simulink model "Model_sim"  (R2024b)
settings: Solver=FixedStepAuto  StartTime=0.0  StopTime=10  FixedStep=0.001  RelTol=1e-3
values from neighbouring files (symbols this model uses):
  A = [      0             1            0         0 ... (first row only)    [QuarterCarModel.m]
  A_Nodamp = [      0             1            0         0 ... (first row only)    [QuarterCarModel.m]
  B = [  0     0     0 ... (first row only)    [QuarterCarModel.m]
  C = [1 0 0 0 ... (first row only)    [QuarterCarModel.m]
  D = zeros(4,3)    [QuarterCarModel.m]
undefined symbols (not defined in the file or in its folder): A_sky, B_sky, c_sky, C_sky, D_sky
settings Model: Creator=elija  LastModifiedBy=elija

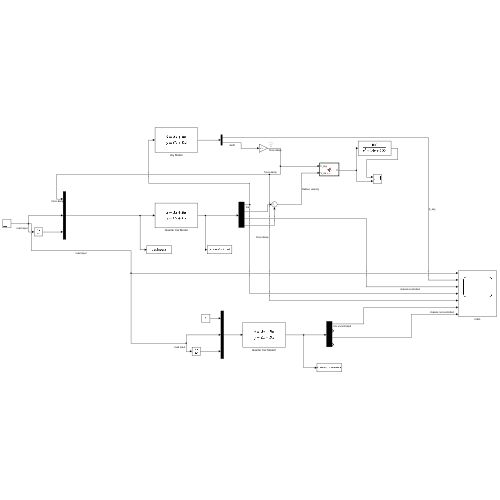
[thumbnail: Simulink's stored preview of the top-level diagram]
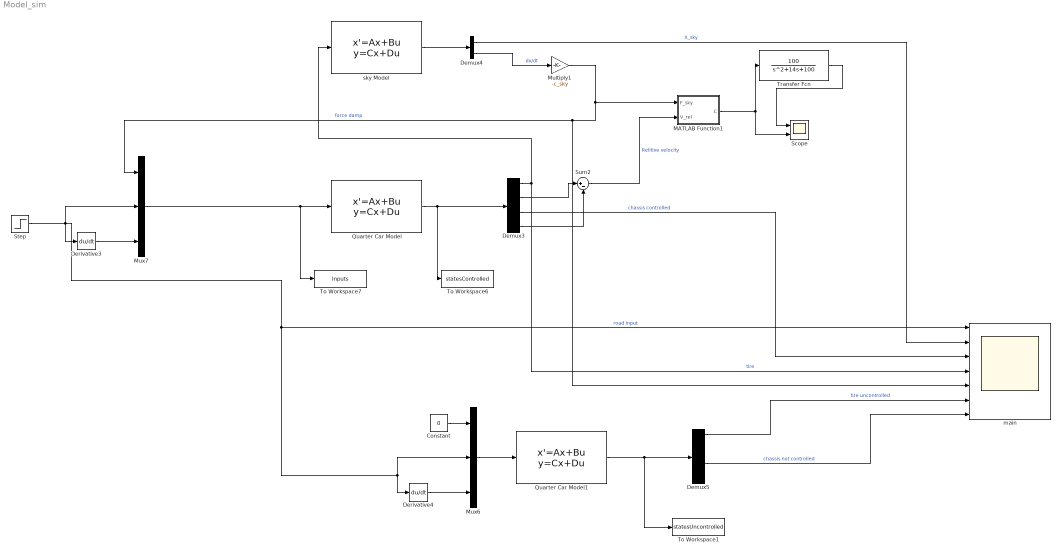
== system Model_sim ==
  Constant : Constant  Value=0
  Demux3 : Demux
  Demux4 : Demux  Outputs=2
  Demux5 : Demux
  Derivative3 : Derivative
  Derivative4 : Derivative
  MATLAB Function1 : MATLAB Function  TreatAsAtomicUnit=on
  Multiply1 : Gain  Gain=-c_sky
  Mux6 : Mux  Inputs=3
  Mux7 : Mux  Inputs=3
  Quarter Car Model : StateSpace  A=A_Nodamp  B=B  C=C  D=D  InitialCondition=0
  Quarter Car Model1 : StateSpace  A=A  B=B  C=C  D=D  InitialCondition=0
  Scope : Scope  NumInputPorts=2
  Step : Step  SampleTime=0
  Sum2 : Sum  Inputs=|+-
  To Workspace1 : ToWorkspace  VariableName=statesUncontrolled  SaveFormat=Timeseries  SampleTime=-1
  To Workspace6 : ToWorkspace  VariableName=statesControlled  SaveFormat=Timeseries  SampleTime=-1
  To Workspace7 : ToWorkspace  VariableName=Inputs  SaveFormat=Timeseries  SampleTime=-1
  Transfer Fcn : TransferFcn  Numerator=[100]  Denominator=[1 14 100]
  main : Scope  NumInputPorts=7
  sky Model : StateSpace  A=A_sky  B=B_sky  C=C_sky  D=D_sky  InitialCondition=0
  wires:
  Step/1 -> Mux6/2, Derivative4/1, main/1, Mux7/2, Derivative3/1  "road input"
  Derivative3/1 -> Mux7/3
  Mux7/1 -> Quarter Car Model/1, To Workspace7/1
  Quarter Car Model/1 -> Demux3/1, To Workspace6/1
  Demux3/1 -> sky Model/1, main/4  "tire"
  Sum2/1 -> MATLAB Function1/2(V_rel)  "Relitive velocity"
  MATLAB Function1/1(C) -> Transfer Fcn/1, Scope/2
  sky Model/1 -> Demux4/1
  Demux4/2 -> Multiply1/1  "dx/dt"
  Demux3/2 -> Sum2/1
  Demux3/4 -> Sum2/2
  Quarter Car Model1/1 -> To Workspace1/1, Demux5/1
  Mux6/1 -> Quarter Car Model1/1
  Derivative4/1 -> Mux6/3
  Demux3/3 -> main/3  "chassis controlled"
  Demux5/3 -> main/7  "chassis not controlled"
  Demux4/1 -> main/2  "X_sky"
  Constant/1 -> Mux6/1
  Transfer Fcn/1 -> Scope/1
  Multiply1/1 -> main/5, Mux7/1, MATLAB Function1/1(F_sky)  "force damp"
  Demux5/1 -> main/6  "tire uncontrolled"

== matlab function Model_sim/MATLAB Function1 ==
  data: F_sky input; V_rel input; C output
function C = fcn(F_sky,V_rel)
C = abs(F_sky)*abs(V_rel);
end
